simulink model "IEEE_13_BUS_Radial"  (R2021b)
settings: Solver=VariableStepAuto  StartTime=0.0  StopTime=48  RelTol=1e-3
undefined symbols (not defined in the file or in its folder): f611, f632, f633, f634, f645, f646, f650, f652, f671, f675, f680, f684, f692
libraries: simulink x416, slpidlib x13
(part 7 of 7)

== system IEEE_13_BUS_Radial/f675/CONTROLLERS/lPoLC2 ==
  Sum : Sum  Inputs=|++
  base : simulink/Sources/Repeating Sequence Stair  OutValues=f675.PoLC2.l  tsamp=f675.PoLC2.ST  OutMin=[]  OutMax=[]  OutDataTypeStr=double  OutputDataTypeScalingMode=double  OutDataType=fixdt(0,8)  ConRadixGroup=Best Precision: Vector-wise  OutScaling=2^-12
  noise : simulink/Sources/Band-Limited White Noise  Cov=f675.PoLC2.Noise  Ts=f675.PoLC2.NoiseST  seed=f675.PoLC2.NoiseSD
  P : Outport  VectorParamsAs1DForOutWhenUnconnected=off
  wires:
  Sum/1 -> P/1
  noise/1 -> Sum/2
  base/1 -> Sum/1

== system IEEE_13_BUS_Radial/f675/CONTROLLERS/lPoLC3 ==
  Sum : Sum  Inputs=|++
  base : simulink/Sources/Repeating Sequence Stair  OutValues=f675.PoLC3.l  tsamp=f675.PoLC3.ST  OutMin=[]  OutMax=[]  OutDataTypeStr=double  OutputDataTypeScalingMode=double  OutDataType=fixdt(0,8)  ConRadixGroup=Best Precision: Vector-wise  OutScaling=2^-12
  noise : simulink/Sources/Band-Limited White Noise  Cov=f675.PoLC3.Noise  Ts=f675.PoLC3.NoiseST  seed=f675.PoLC3.NoiseSD
  P : Outport  VectorParamsAs1DForOutWhenUnconnected=off
  wires:
  Sum/1 -> P/1
  noise/1 -> Sum/2
  base/1 -> Sum/1

== system IEEE_13_BUS_Radial/f675/CONTROLLERS/lPoLC4 ==
  Sum : Sum  Inputs=|++
  base : simulink/Sources/Repeating Sequence Stair  OutValues=f675.PoLC4.l  tsamp=f675.PoLC4.ST  OutMin=[]  OutMax=[]  OutDataTypeStr=double  OutputDataTypeScalingMode=double  OutDataType=fixdt(0,8)  ConRadixGroup=Best Precision: Vector-wise  OutScaling=2^-12
  noise : simulink/Sources/Band-Limited White Noise  Cov=f675.PoLC4.Noise  Ts=f675.PoLC4.NoiseST  seed=f675.PoLC4.NoiseSD
  P : Outport  VectorParamsAs1DForOutWhenUnconnected=off
  wires:
  Sum/1 -> P/1
  noise/1 -> Sum/2
  base/1 -> Sum/1

== system IEEE_13_BUS_Radial/f675/CONTROLLERS/lPoLC5 ==
  Sum : Sum  Inputs=|++
  base : simulink/Sources/Repeating Sequence Stair  OutValues=f675.PoLC5.l  tsamp=f675.PoLC5.ST  OutMin=[]  OutMax=[]  OutDataTypeStr=double  OutputDataTypeScalingMode=double  OutDataType=fixdt(0,8)  ConRadixGroup=Best Precision: Vector-wise  OutScaling=2^-12
  noise : simulink/Sources/Band-Limited White Noise  Cov=f675.PoLC5.Noise  Ts=f675.PoLC5.NoiseST  seed=f675.PoLC5.NoiseSD
  P : Outport  VectorParamsAs1DForOutWhenUnconnected=off
  wires:
  Sum/1 -> P/1
  noise/1 -> Sum/2
  base/1 -> Sum/1

== system IEEE_13_BUS_Radial/f675/CONTROLLERS/lPoLC6 ==
  Sum : Sum  Inputs=|++
  base : simulink/Sources/Repeating Sequence Stair  OutValues=f675.PoLC6.l  tsamp=f675.PoLC6.ST  OutMin=[]  OutMax=[]  OutDataTypeStr=double  OutputDataTypeScalingMode=double  OutDataType=fixdt(0,8)  ConRadixGroup=Best Precision: Vector-wise  OutScaling=2^-12
  noise : simulink/Sources/Band-Limited White Noise  Cov=f675.PoLC6.Noise  Ts=f675.PoLC6.NoiseST  seed=f675.PoLC6.NoiseSD
  P : Outport  VectorParamsAs1DForOutWhenUnconnected=off
  wires:
  Sum/1 -> P/1
  noise/1 -> Sum/2
  base/1 -> Sum/1

== system IEEE_13_BUS_Radial/f675/CONTROLLERS/lPoLC7 ==
  Sum : Sum  Inputs=|++
  base : simulink/Sources/Repeating Sequence Stair  OutValues=f675.PoLC7.l  tsamp=f675.PoLC7.ST  OutMin=[]  OutMax=[]  OutDataTypeStr=double  OutputDataTypeScalingMode=double  OutDataType=fixdt(0,8)  ConRadixGroup=Best Precision: Vector-wise  OutScaling=2^-12
  noise : simulink/Sources/Band-Limited White Noise  Cov=f675.PoLC7.Noise  Ts=f675.PoLC7.NoiseST  seed=f675.PoLC7.NoiseSD
  P : Outport  VectorParamsAs1DForOutWhenUnconnected=off
  wires:
  Sum/1 -> P/1
  noise/1 -> Sum/2
  base/1 -> Sum/1

== system IEEE_13_BUS_Radial/f675/CONTROLLERS/lPoLC8 ==
  Sum : Sum  Inputs=|++
  base : simulink/Sources/Repeating Sequence Stair  OutValues=f675.PoLC8.l  tsamp=f675.PoLC8.ST  OutMin=[]  OutMax=[]  OutDataTypeStr=double  OutputDataTypeScalingMode=double  OutDataType=fixdt(0,8)  ConRadixGroup=Best Precision: Vector-wise  OutScaling=2^-12
  noise : simulink/Sources/Band-Limited White Noise  Cov=f675.PoLC8.Noise  Ts=f675.PoLC8.NoiseST  seed=f675.PoLC8.NoiseSD
  P : Outport  VectorParamsAs1DForOutWhenUnconnected=off
  wires:
  Sum/1 -> P/1
  noise/1 -> Sum/2
  base/1 -> Sum/1

== system IEEE_13_BUS_Radial/f675/CONTROLLERS/lPoLC9 ==
  Sum : Sum  Inputs=|++
  base : simulink/Sources/Repeating Sequence Stair  OutValues=f675.PoLC9.l  tsamp=f675.PoLC9.ST  OutMin=[]  OutMax=[]  OutDataTypeStr=double  OutputDataTypeScalingMode=double  OutDataType=fixdt(0,8)  ConRadixGroup=Best Precision: Vector-wise  OutScaling=2^-12
  noise : simulink/Sources/Band-Limited White Noise  Cov=f675.PoLC9.Noise  Ts=f675.PoLC9.NoiseST  seed=f675.PoLC9.NoiseSD
  P : Outport  VectorParamsAs1DForOutWhenUnconnected=off
  wires:
  Sum/1 -> P/1
  noise/1 -> Sum/2
  base/1 -> Sum/1

== system IEEE_13_BUS_Radial/f675/OPERATIONS GATEWAY/Agent Communications ==
  Enable : EnablePort
  Constant : Constant  Value=0
  Out1 : Outport  VectorParamsAs1DForOutWhenUnconnected=off
  wires:
  Constant/1 -> Out1/1

== system IEEE_13_BUS_Radial/f680/CONTROLLERS/lPoLC1 ==
  Sum : Sum  Inputs=|++
  base : simulink/Sources/Repeating Sequence Stair  OutValues=f680.PoLC1.l  tsamp=f680.PoLC1.ST  OutMin=[]  OutMax=[]  OutDataTypeStr=double  OutputDataTypeScalingMode=double  OutDataType=fixdt(0,8)  ConRadixGroup=Best Precision: Vector-wise  OutScaling=2^-12
  noise : simulink/Sources/Band-Limited White Noise  Cov=f680.PoLC1.Noise  Ts=f680.PoLC1.NoiseST  seed=f680.PoLC1.NoiseSD
  P : Outport  VectorParamsAs1DForOutWhenUnconnected=off
  wires:
  Sum/1 -> P/1
  noise/1 -> Sum/2
  base/1 -> Sum/1

== system IEEE_13_BUS_Radial/f680/CONTROLLERS/lPoLC10 ==
  Sum : Sum  Inputs=|++
  base : simulink/Sources/Repeating Sequence Stair  OutValues=f680.PoLC10.l  tsamp=f680.PoLC10.ST  OutMin=[]  OutMax=[]  OutDataTypeStr=double  OutputDataTypeScalingMode=double  OutDataType=fixdt(0,8)  ConRadixGroup=Best Precision: Vector-wise  OutScaling=2^-12
  noise : simulink/Sources/Band-Limited White Noise  Cov=f680.PoLC10.Noise  Ts=f680.PoLC10.NoiseST  seed=f680.PoLC10.NoiseSD
  P : Outport  VectorParamsAs1DForOutWhenUnconnected=off
  wires:
  Sum/1 -> P/1
  noise/1 -> Sum/2
  base/1 -> Sum/1

== system IEEE_13_BUS_Radial/f680/CONTROLLERS/lPoLC11 ==
  Sum : Sum  Inputs=|++
  base : simulink/Sources/Repeating Sequence Stair  OutValues=f680.PoLC11.l  tsamp=f680.PoLC11.ST  OutMin=[]  OutMax=[]  OutDataTypeStr=double  OutputDataTypeScalingMode=double  OutDataType=fixdt(0,8)  ConRadixGroup=Best Precision: Vector-wise  OutScaling=2^-12
  noise : simulink/Sources/Band-Limited White Noise  Cov=f680.PoLC11.Noise  Ts=f680.PoLC11.NoiseST  seed=f680.PoLC11.NoiseSD
  P : Outport  VectorParamsAs1DForOutWhenUnconnected=off
  wires:
  Sum/1 -> P/1
  noise/1 -> Sum/2
  base/1 -> Sum/1

== system IEEE_13_BUS_Radial/f680/CONTROLLERS/lPoLC12 ==
  Sum : Sum  Inputs=|++
  base : simulink/Sources/Repeating Sequence Stair  OutValues=f680.PoLC12.l  tsamp=f680.PoLC12.ST  OutMin=[]  OutMax=[]  OutDataTypeStr=double  OutputDataTypeScalingMode=double  OutDataType=fixdt(0,8)  ConRadixGroup=Best Precision: Vector-wise  OutScaling=2^-12
  noise : simulink/Sources/Band-Limited White Noise  Cov=f680.PoLC12.Noise  Ts=f680.PoLC12.NoiseST  seed=f680.PoLC12.NoiseSD
  P : Outport  VectorParamsAs1DForOutWhenUnconnected=off
  wires:
  Sum/1 -> P/1
  noise/1 -> Sum/2
  base/1 -> Sum/1

== system IEEE_13_BUS_Radial/f680/CONTROLLERS/lPoLC13 ==
  Sum : Sum  Inputs=|++
  base : simulink/Sources/Repeating Sequence Stair  OutValues=f680.PoLC13.l  tsamp=f680.PoLC13.ST  OutMin=[]  OutMax=[]  OutDataTypeStr=double  OutputDataTypeScalingMode=double  OutDataType=fixdt(0,8)  ConRadixGroup=Best Precision: Vector-wise  OutScaling=2^-12
  noise : simulink/Sources/Band-Limited White Noise  Cov=f680.PoLC13.Noise  Ts=f680.PoLC13.NoiseST  seed=f680.PoLC13.NoiseSD
  P : Outport  VectorParamsAs1DForOutWhenUnconnected=off
  wires:
  Sum/1 -> P/1
  noise/1 -> Sum/2
  base/1 -> Sum/1

== system IEEE_13_BUS_Radial/f680/CONTROLLERS/lPoLC14 ==
  Sum : Sum  Inputs=|++
  base : simulink/Sources/Repeating Sequence Stair  OutValues=f680.PoLC14.l  tsamp=f680.PoLC14.ST  OutMin=[]  OutMax=[]  OutDataTypeStr=double  OutputDataTypeScalingMode=double  OutDataType=fixdt(0,8)  ConRadixGroup=Best Precision: Vector-wise  OutScaling=2^-12
  noise : simulink/Sources/Band-Limited White Noise  Cov=f680.PoLC14.Noise  Ts=f680.PoLC14.NoiseST  seed=f680.PoLC14.NoiseSD
  P : Outport  VectorParamsAs1DForOutWhenUnconnected=off
  wires:
  Sum/1 -> P/1
  noise/1 -> Sum/2
  base/1 -> Sum/1

== system IEEE_13_BUS_Radial/f680/CONTROLLERS/lPoLC15 ==
  Sum : Sum  Inputs=|++
  base : simulink/Sources/Repeating Sequence Stair  OutValues=f680.PoLC15.l  tsamp=f680.PoLC15.ST  OutMin=[]  OutMax=[]  OutDataTypeStr=double  OutputDataTypeScalingMode=double  OutDataType=fixdt(0,8)  ConRadixGroup=Best Precision: Vector-wise  OutScaling=2^-12
  noise : simulink/Sources/Band-Limited White Noise  Cov=f680.PoLC15.Noise  Ts=f680.PoLC15.NoiseST  seed=f680.PoLC15.NoiseSD
  P : Outport  VectorParamsAs1DForOutWhenUnconnected=off
  wires:
  Sum/1 -> P/1
  noise/1 -> Sum/2
  base/1 -> Sum/1

== system IEEE_13_BUS_Radial/f680/CONTROLLERS/lPoLC16 ==
  cv : Inport
  Sum : Sum  Inputs=|++
  Terminator : Terminator
  base : simulink/Sources/Repeating Sequence Stair  OutValues=f680.PoLC16.l  tsamp=f680.PoLC16.ST  OutMin=[]  OutMax=[]  OutDataTypeStr=double  OutputDataTypeScalingMode=double  OutDataType=fixdt(0,8)  ConRadixGroup=Best Precision: Vector-wise  OutScaling=2^-12
  noise : simulink/Sources/Band-Limited White Noise  Cov=f680.PoLC16.Noise  Ts=f680.PoLC16.NoiseST  seed=f680.PoLC16.NoiseSD
  P : Outport  VectorParamsAs1DForOutWhenUnconnected=off
  wires:
  Sum/1 -> Terminator/1
  noise/1 -> Sum/2
  base/1 -> Sum/1
  cv/1 -> P/1

== system IEEE_13_BUS_Radial/f680/CONTROLLERS/lPoLC2 ==
  Sum : Sum  Inputs=|++
  base : simulink/Sources/Repeating Sequence Stair  OutValues=f680.PoLC2.l  tsamp=f680.PoLC2.ST  OutMin=[]  OutMax=[]  OutDataTypeStr=double  OutputDataTypeScalingMode=double  OutDataType=fixdt(0,8)  ConRadixGroup=Best Precision: Vector-wise  OutScaling=2^-12
  noise : simulink/Sources/Band-Limited White Noise  Cov=f680.PoLC2.Noise  Ts=f680.PoLC2.NoiseST  seed=f680.PoLC2.NoiseSD
  P : Outport  VectorParamsAs1DForOutWhenUnconnected=off
  wires:
  Sum/1 -> P/1
  noise/1 -> Sum/2
  base/1 -> Sum/1

== system IEEE_13_BUS_Radial/f680/CONTROLLERS/lPoLC3 ==
  Sum : Sum  Inputs=|++
  base : simulink/Sources/Repeating Sequence Stair  OutValues=f680.PoLC3.l  tsamp=f680.PoLC3.ST  OutMin=[]  OutMax=[]  OutDataTypeStr=double  OutputDataTypeScalingMode=double  OutDataType=fixdt(0,8)  ConRadixGroup=Best Precision: Vector-wise  OutScaling=2^-12
  noise : simulink/Sources/Band-Limited White Noise  Cov=f680.PoLC3.Noise  Ts=f680.PoLC3.NoiseST  seed=f680.PoLC3.NoiseSD
  P : Outport  VectorParamsAs1DForOutWhenUnconnected=off
  wires:
  Sum/1 -> P/1
  noise/1 -> Sum/2
  base/1 -> Sum/1

== system IEEE_13_BUS_Radial/f680/CONTROLLERS/lPoLC4 ==
  Sum : Sum  Inputs=|++
  base : simulink/Sources/Repeating Sequence Stair  OutValues=f680.PoLC4.l  tsamp=f680.PoLC4.ST  OutMin=[]  OutMax=[]  OutDataTypeStr=double  OutputDataTypeScalingMode=double  OutDataType=fixdt(0,8)  ConRadixGroup=Best Precision: Vector-wise  OutScaling=2^-12
  noise : simulink/Sources/Band-Limited White Noise  Cov=f680.PoLC4.Noise  Ts=f680.PoLC4.NoiseST  seed=f680.PoLC4.NoiseSD
  P : Outport  VectorParamsAs1DForOutWhenUnconnected=off
  wires:
  Sum/1 -> P/1
  noise/1 -> Sum/2
  base/1 -> Sum/1

== system IEEE_13_BUS_Radial/f680/CONTROLLERS/lPoLC5 ==
  Sum : Sum  Inputs=|++
  base : simulink/Sources/Repeating Sequence Stair  OutValues=f680.PoLC5.l  tsamp=f680.PoLC5.ST  OutMin=[]  OutMax=[]  OutDataTypeStr=double  OutputDataTypeScalingMode=double  OutDataType=fixdt(0,8)  ConRadixGroup=Best Precision: Vector-wise  OutScaling=2^-12
  noise : simulink/Sources/Band-Limited White Noise  Cov=f680.PoLC5.Noise  Ts=f680.PoLC5.NoiseST  seed=f680.PoLC5.NoiseSD
  P : Outport  VectorParamsAs1DForOutWhenUnconnected=off
  wires:
  Sum/1 -> P/1
  noise/1 -> Sum/2
  base/1 -> Sum/1

== system IEEE_13_BUS_Radial/f680/CONTROLLERS/lPoLC6 ==
  Sum : Sum  Inputs=|++
  base : simulink/Sources/Repeating Sequence Stair  OutValues=f680.PoLC6.l  tsamp=f680.PoLC6.ST  OutMin=[]  OutMax=[]  OutDataTypeStr=double  OutputDataTypeScalingMode=double  OutDataType=fixdt(0,8)  ConRadixGroup=Best Precision: Vector-wise  OutScaling=2^-12
  noise : simulink/Sources/Band-Limited White Noise  Cov=f680.PoLC6.Noise  Ts=f680.PoLC6.NoiseST  seed=f680.PoLC6.NoiseSD
  P : Outport  VectorParamsAs1DForOutWhenUnconnected=off
  wires:
  Sum/1 -> P/1
  noise/1 -> Sum/2
  base/1 -> Sum/1

== system IEEE_13_BUS_Radial/f680/CONTROLLERS/lPoLC7 ==
  Sum : Sum  Inputs=|++
  base : simulink/Sources/Repeating Sequence Stair  OutValues=f680.PoLC7.l  tsamp=f680.PoLC7.ST  OutMin=[]  OutMax=[]  OutDataTypeStr=double  OutputDataTypeScalingMode=double  OutDataType=fixdt(0,8)  ConRadixGroup=Best Precision: Vector-wise  OutScaling=2^-12
  noise : simulink/Sources/Band-Limited White Noise  Cov=f680.PoLC7.Noise  Ts=f680.PoLC7.NoiseST  seed=f680.PoLC7.NoiseSD
  P : Outport  VectorParamsAs1DForOutWhenUnconnected=off
  wires:
  Sum/1 -> P/1
  noise/1 -> Sum/2
  base/1 -> Sum/1

== system IEEE_13_BUS_Radial/f680/CONTROLLERS/lPoLC8 ==
  Sum : Sum  Inputs=|++
  base : simulink/Sources/Repeating Sequence Stair  OutValues=f680.PoLC8.l  tsamp=f680.PoLC8.ST  OutMin=[]  OutMax=[]  OutDataTypeStr=double  OutputDataTypeScalingMode=double  OutDataType=fixdt(0,8)  ConRadixGroup=Best Precision: Vector-wise  OutScaling=2^-12
  noise : simulink/Sources/Band-Limited White Noise  Cov=f680.PoLC8.Noise  Ts=f680.PoLC8.NoiseST  seed=f680.PoLC8.NoiseSD
  P : Outport  VectorParamsAs1DForOutWhenUnconnected=off
  wires:
  Sum/1 -> P/1
  noise/1 -> Sum/2
  base/1 -> Sum/1

== system IEEE_13_BUS_Radial/f680/CONTROLLERS/lPoLC9 ==
  Sum : Sum  Inputs=|++
  base : simulink/Sources/Repeating Sequence Stair  OutValues=f680.PoLC9.l  tsamp=f680.PoLC9.ST  OutMin=[]  OutMax=[]  OutDataTypeStr=double  OutputDataTypeScalingMode=double  OutDataType=fixdt(0,8)  ConRadixGroup=Best Precision: Vector-wise  OutScaling=2^-12
  noise : simulink/Sources/Band-Limited White Noise  Cov=f680.PoLC9.Noise  Ts=f680.PoLC9.NoiseST  seed=f680.PoLC9.NoiseSD
  P : Outport  VectorParamsAs1DForOutWhenUnconnected=off
  wires:
  Sum/1 -> P/1
  noise/1 -> Sum/2
  base/1 -> Sum/1

== system IEEE_13_BUS_Radial/f680/OPERATIONS GATEWAY/Agent Communications ==
  Enable : EnablePort
  Constant : Constant  Value=0
  Out1 : Outport  VectorParamsAs1DForOutWhenUnconnected=off
  wires:
  Constant/1 -> Out1/1

== system IEEE_13_BUS_Radial/f684/CONTROLLERS/lPoLC1 ==
  Sum : Sum  Inputs=|++
  base : simulink/Sources/Repeating Sequence Stair  OutValues=f684.PoLC1.l  tsamp=f684.PoLC1.ST  OutMin=[]  OutMax=[]  OutDataTypeStr=double  OutputDataTypeScalingMode=double  OutDataType=fixdt(0,8)  ConRadixGroup=Best Precision: Vector-wise  OutScaling=2^-12
  noise : simulink/Sources/Band-Limited White Noise  Cov=f684.PoLC1.Noise  Ts=f684.PoLC1.NoiseST  seed=f684.PoLC1.NoiseSD
  P : Outport  VectorParamsAs1DForOutWhenUnconnected=off
  wires:
  Sum/1 -> P/1
  noise/1 -> Sum/2
  base/1 -> Sum/1

== system IEEE_13_BUS_Radial/f684/CONTROLLERS/lPoLC10 ==
  Sum : Sum  Inputs=|++
  base : simulink/Sources/Repeating Sequence Stair  OutValues=f684.PoLC10.l  tsamp=f684.PoLC10.ST  OutMin=[]  OutMax=[]  OutDataTypeStr=double  OutputDataTypeScalingMode=double  OutDataType=fixdt(0,8)  ConRadixGroup=Best Precision: Vector-wise  OutScaling=2^-12
  noise : simulink/Sources/Band-Limited White Noise  Cov=f684.PoLC10.Noise  Ts=f684.PoLC10.NoiseST  seed=f684.PoLC10.NoiseSD
  P : Outport  VectorParamsAs1DForOutWhenUnconnected=off
  wires:
  Sum/1 -> P/1
  noise/1 -> Sum/2
  base/1 -> Sum/1

== system IEEE_13_BUS_Radial/f684/CONTROLLERS/lPoLC11 ==
  Sum : Sum  Inputs=|++
  base : simulink/Sources/Repeating Sequence Stair  OutValues=f684.PoLC11.l  tsamp=f684.PoLC11.ST  OutMin=[]  OutMax=[]  OutDataTypeStr=double  OutputDataTypeScalingMode=double  OutDataType=fixdt(0,8)  ConRadixGroup=Best Precision: Vector-wise  OutScaling=2^-12
  noise : simulink/Sources/Band-Limited White Noise  Cov=f684.PoLC11.Noise  Ts=f684.PoLC11.NoiseST  seed=f684.PoLC11.NoiseSD
  P : Outport  VectorParamsAs1DForOutWhenUnconnected=off
  wires:
  Sum/1 -> P/1
  noise/1 -> Sum/2
  base/1 -> Sum/1

== system IEEE_13_BUS_Radial/f684/CONTROLLERS/lPoLC12 ==
  Sum : Sum  Inputs=|++
  base : simulink/Sources/Repeating Sequence Stair  OutValues=f684.PoLC12.l  tsamp=f684.PoLC12.ST  OutMin=[]  OutMax=[]  OutDataTypeStr=double  OutputDataTypeScalingMode=double  OutDataType=fixdt(0,8)  ConRadixGroup=Best Precision: Vector-wise  OutScaling=2^-12
  noise : simulink/Sources/Band-Limited White Noise  Cov=f684.PoLC12.Noise  Ts=f684.PoLC12.NoiseST  seed=f684.PoLC12.NoiseSD
  P : Outport  VectorParamsAs1DForOutWhenUnconnected=off
  wires:
  Sum/1 -> P/1
  noise/1 -> Sum/2
  base/1 -> Sum/1

== system IEEE_13_BUS_Radial/f684/CONTROLLERS/lPoLC13 ==
  Sum : Sum  Inputs=|++
  base : simulink/Sources/Repeating Sequence Stair  OutValues=f684.PoLC13.l  tsamp=f684.PoLC13.ST  OutMin=[]  OutMax=[]  OutDataTypeStr=double  OutputDataTypeScalingMode=double  OutDataType=fixdt(0,8)  ConRadixGroup=Best Precision: Vector-wise  OutScaling=2^-12
  noise : simulink/Sources/Band-Limited White Noise  Cov=f684.PoLC13.Noise  Ts=f684.PoLC13.NoiseST  seed=f684.PoLC13.NoiseSD
  P : Outport  VectorParamsAs1DForOutWhenUnconnected=off
  wires:
  Sum/1 -> P/1
  noise/1 -> Sum/2
  base/1 -> Sum/1

== system IEEE_13_BUS_Radial/f684/CONTROLLERS/lPoLC14 ==
  Sum : Sum  Inputs=|++
  base : simulink/Sources/Repeating Sequence Stair  OutValues=f684.PoLC14.l  tsamp=f684.PoLC14.ST  OutMin=[]  OutMax=[]  OutDataTypeStr=double  OutputDataTypeScalingMode=double  OutDataType=fixdt(0,8)  ConRadixGroup=Best Precision: Vector-wise  OutScaling=2^-12
  noise : simulink/Sources/Band-Limited White Noise  Cov=f684.PoLC14.Noise  Ts=f684.PoLC14.NoiseST  seed=f684.PoLC14.NoiseSD
  P : Outport  VectorParamsAs1DForOutWhenUnconnected=off
  wires:
  Sum/1 -> P/1
  noise/1 -> Sum/2
  base/1 -> Sum/1

== system IEEE_13_BUS_Radial/f684/CONTROLLERS/lPoLC15 ==
  Sum : Sum  Inputs=|++
  base : simulink/Sources/Repeating Sequence Stair  OutValues=f684.PoLC15.l  tsamp=f684.PoLC15.ST  OutMin=[]  OutMax=[]  OutDataTypeStr=double  OutputDataTypeScalingMode=double  OutDataType=fixdt(0,8)  ConRadixGroup=Best Precision: Vector-wise  OutScaling=2^-12
  noise : simulink/Sources/Band-Limited White Noise  Cov=f684.PoLC15.Noise  Ts=f684.PoLC15.NoiseST  seed=f684.PoLC15.NoiseSD
  P : Outport  VectorParamsAs1DForOutWhenUnconnected=off
  wires:
  Sum/1 -> P/1
  noise/1 -> Sum/2
  base/1 -> Sum/1

== system IEEE_13_BUS_Radial/f684/CONTROLLERS/lPoLC16 ==
  cv : Inport
  Sum : Sum  Inputs=|++
  Terminator : Terminator
  base : simulink/Sources/Repeating Sequence Stair  OutValues=f684.PoLC16.l  tsamp=f684.PoLC16.ST  OutMin=[]  OutMax=[]  OutDataTypeStr=double  OutputDataTypeScalingMode=double  OutDataType=fixdt(0,8)  ConRadixGroup=Best Precision: Vector-wise  OutScaling=2^-12
  noise : simulink/Sources/Band-Limited White Noise  Cov=f684.PoLC16.Noise  Ts=f684.PoLC16.NoiseST  seed=f684.PoLC16.NoiseSD
  P : Outport  VectorParamsAs1DForOutWhenUnconnected=off
  wires:
  Sum/1 -> Terminator/1
  noise/1 -> Sum/2
  base/1 -> Sum/1
  cv/1 -> P/1

== system IEEE_13_BUS_Radial/f684/CONTROLLERS/lPoLC2 ==
  Sum : Sum  Inputs=|++
  base : simulink/Sources/Repeating Sequence Stair  OutValues=f684.PoLC2.l  tsamp=f684.PoLC2.ST  OutMin=[]  OutMax=[]  OutDataTypeStr=double  OutputDataTypeScalingMode=double  OutDataType=fixdt(0,8)  ConRadixGroup=Best Precision: Vector-wise  OutScaling=2^-12
  noise : simulink/Sources/Band-Limited White Noise  Cov=f684.PoLC2.Noise  Ts=f684.PoLC2.NoiseST  seed=f684.PoLC2.NoiseSD
  P : Outport  VectorParamsAs1DForOutWhenUnconnected=off
  wires:
  Sum/1 -> P/1
  noise/1 -> Sum/2
  base/1 -> Sum/1

== system IEEE_13_BUS_Radial/f684/CONTROLLERS/lPoLC3 ==
  Sum : Sum  Inputs=|++
  base : simulink/Sources/Repeating Sequence Stair  OutValues=f684.PoLC3.l  tsamp=f684.PoLC3.ST  OutMin=[]  OutMax=[]  OutDataTypeStr=double  OutputDataTypeScalingMode=double  OutDataType=fixdt(0,8)  ConRadixGroup=Best Precision: Vector-wise  OutScaling=2^-12
  noise : simulink/Sources/Band-Limited White Noise  Cov=f684.PoLC3.Noise  Ts=f684.PoLC3.NoiseST  seed=f684.PoLC3.NoiseSD
  P : Outport  VectorParamsAs1DForOutWhenUnconnected=off
  wires:
  Sum/1 -> P/1
  noise/1 -> Sum/2
  base/1 -> Sum/1

== system IEEE_13_BUS_Radial/f684/CONTROLLERS/lPoLC4 ==
  Sum : Sum  Inputs=|++
  base : simulink/Sources/Repeating Sequence Stair  OutValues=f684.PoLC4.l  tsamp=f684.PoLC4.ST  OutMin=[]  OutMax=[]  OutDataTypeStr=double  OutputDataTypeScalingMode=double  OutDataType=fixdt(0,8)  ConRadixGroup=Best Precision: Vector-wise  OutScaling=2^-12
  noise : simulink/Sources/Band-Limited White Noise  Cov=f684.PoLC4.Noise  Ts=f684.PoLC4.NoiseST  seed=f684.PoLC4.NoiseSD
  P : Outport  VectorParamsAs1DForOutWhenUnconnected=off
  wires:
  Sum/1 -> P/1
  noise/1 -> Sum/2
  base/1 -> Sum/1

== system IEEE_13_BUS_Radial/f684/CONTROLLERS/lPoLC5 ==
  Sum : Sum  Inputs=|++
  base : simulink/Sources/Repeating Sequence Stair  OutValues=f684.PoLC5.l  tsamp=f684.PoLC5.ST  OutMin=[]  OutMax=[]  OutDataTypeStr=double  OutputDataTypeScalingMode=double  OutDataType=fixdt(0,8)  ConRadixGroup=Best Precision: Vector-wise  OutScaling=2^-12
  noise : simulink/Sources/Band-Limited White Noise  Cov=f684.PoLC5.Noise  Ts=f684.PoLC5.NoiseST  seed=f684.PoLC5.NoiseSD
  P : Outport  VectorParamsAs1DForOutWhenUnconnected=off
  wires:
  Sum/1 -> P/1
  noise/1 -> Sum/2
  base/1 -> Sum/1

== system IEEE_13_BUS_Radial/f684/CONTROLLERS/lPoLC6 ==
  Sum : Sum  Inputs=|++
  base : simulink/Sources/Repeating Sequence Stair  OutValues=f684.PoLC6.l  tsamp=f684.PoLC6.ST  OutMin=[]  OutMax=[]  OutDataTypeStr=double  OutputDataTypeScalingMode=double  OutDataType=fixdt(0,8)  ConRadixGroup=Best Precision: Vector-wise  OutScaling=2^-12
  noise : simulink/Sources/Band-Limited White Noise  Cov=f684.PoLC6.Noise  Ts=f684.PoLC6.NoiseST  seed=f684.PoLC6.NoiseSD
  P : Outport  VectorParamsAs1DForOutWhenUnconnected=off
  wires:
  Sum/1 -> P/1
  noise/1 -> Sum/2
  base/1 -> Sum/1

== system IEEE_13_BUS_Radial/f684/CONTROLLERS/lPoLC7 ==
  Sum : Sum  Inputs=|++
  base : simulink/Sources/Repeating Sequence Stair  OutValues=f684.PoLC7.l  tsamp=f684.PoLC7.ST  OutMin=[]  OutMax=[]  OutDataTypeStr=double  OutputDataTypeScalingMode=double  OutDataType=fixdt(0,8)  ConRadixGroup=Best Precision: Vector-wise  OutScaling=2^-12
  noise : simulink/Sources/Band-Limited White Noise  Cov=f684.PoLC7.Noise  Ts=f684.PoLC7.NoiseST  seed=f684.PoLC7.NoiseSD
  P : Outport  VectorParamsAs1DForOutWhenUnconnected=off
  wires:
  Sum/1 -> P/1
  noise/1 -> Sum/2
  base/1 -> Sum/1

== system IEEE_13_BUS_Radial/f684/CONTROLLERS/lPoLC8 ==
  Sum : Sum  Inputs=|++
  base : simulink/Sources/Repeating Sequence Stair  OutValues=f684.PoLC8.l  tsamp=f684.PoLC8.ST  OutMin=[]  OutMax=[]  OutDataTypeStr=double  OutputDataTypeScalingMode=double  OutDataType=fixdt(0,8)  ConRadixGroup=Best Precision: Vector-wise  OutScaling=2^-12
  noise : simulink/Sources/Band-Limited White Noise  Cov=f684.PoLC8.Noise  Ts=f684.PoLC8.NoiseST  seed=f684.PoLC8.NoiseSD
  P : Outport  VectorParamsAs1DForOutWhenUnconnected=off
  wires:
  Sum/1 -> P/1
  noise/1 -> Sum/2
  base/1 -> Sum/1

== system IEEE_13_BUS_Radial/f684/CONTROLLERS/lPoLC9 ==
  Sum : Sum  Inputs=|++
  base : simulink/Sources/Repeating Sequence Stair  OutValues=f684.PoLC9.l  tsamp=f684.PoLC9.ST  OutMin=[]  OutMax=[]  OutDataTypeStr=double  OutputDataTypeScalingMode=double  OutDataType=fixdt(0,8)  ConRadixGroup=Best Precision: Vector-wise  OutScaling=2^-12
  noise : simulink/Sources/Band-Limited White Noise  Cov=f684.PoLC9.Noise  Ts=f684.PoLC9.NoiseST  seed=f684.PoLC9.NoiseSD
  P : Outport  VectorParamsAs1DForOutWhenUnconnected=off
  wires:
  Sum/1 -> P/1
  noise/1 -> Sum/2
  base/1 -> Sum/1

== system IEEE_13_BUS_Radial/f684/OPERATIONS GATEWAY/Agent Communications ==
  Enable : EnablePort
  Constant : Constant  Value=0
  Out1 : Outport  VectorParamsAs1DForOutWhenUnconnected=off
  wires:
  Constant/1 -> Out1/1

== system IEEE_13_BUS_Radial/f692/CONTROLLERS/lPoLC1 ==
  Sum : Sum  Inputs=|++
  base : simulink/Sources/Repeating Sequence Stair  OutValues=f692.PoLC1.l  tsamp=f692.PoLC1.ST  OutMin=[]  OutMax=[]  OutDataTypeStr=double  OutputDataTypeScalingMode=double  OutDataType=fixdt(0,8)  ConRadixGroup=Best Precision: Vector-wise  OutScaling=2^-12
  noise : simulink/Sources/Band-Limited White Noise  Cov=f692.PoLC1.Noise  Ts=f692.PoLC1.NoiseST  seed=f692.PoLC1.NoiseSD
  P : Outport  VectorParamsAs1DForOutWhenUnconnected=off
  wires:
  Sum/1 -> P/1
  noise/1 -> Sum/2
  base/1 -> Sum/1

== system IEEE_13_BUS_Radial/f692/CONTROLLERS/lPoLC10 ==
  Sum : Sum  Inputs=|++
  base : simulink/Sources/Repeating Sequence Stair  OutValues=f692.PoLC10.l  tsamp=f692.PoLC10.ST  OutMin=[]  OutMax=[]  OutDataTypeStr=double  OutputDataTypeScalingMode=double  OutDataType=fixdt(0,8)  ConRadixGroup=Best Precision: Vector-wise  OutScaling=2^-12
  noise : simulink/Sources/Band-Limited White Noise  Cov=f692.PoLC10.Noise  Ts=f692.PoLC10.NoiseST  seed=f692.PoLC10.NoiseSD
  P : Outport  VectorParamsAs1DForOutWhenUnconnected=off
  wires:
  Sum/1 -> P/1
  noise/1 -> Sum/2
  base/1 -> Sum/1

== system IEEE_13_BUS_Radial/f692/CONTROLLERS/lPoLC11 ==
  Sum : Sum  Inputs=|++
  base : simulink/Sources/Repeating Sequence Stair  OutValues=f692.PoLC11.l  tsamp=f692.PoLC11.ST  OutMin=[]  OutMax=[]  OutDataTypeStr=double  OutputDataTypeScalingMode=double  OutDataType=fixdt(0,8)  ConRadixGroup=Best Precision: Vector-wise  OutScaling=2^-12
  noise : simulink/Sources/Band-Limited White Noise  Cov=f692.PoLC11.Noise  Ts=f692.PoLC11.NoiseST  seed=f692.PoLC11.NoiseSD
  P : Outport  VectorParamsAs1DForOutWhenUnconnected=off
  wires:
  Sum/1 -> P/1
  noise/1 -> Sum/2
  base/1 -> Sum/1

== system IEEE_13_BUS_Radial/f692/CONTROLLERS/lPoLC12 ==
  Sum : Sum  Inputs=|++
  base : simulink/Sources/Repeating Sequence Stair  OutValues=f692.PoLC12.l  tsamp=f692.PoLC12.ST  OutMin=[]  OutMax=[]  OutDataTypeStr=double  OutputDataTypeScalingMode=double  OutDataType=fixdt(0,8)  ConRadixGroup=Best Precision: Vector-wise  OutScaling=2^-12
  noise : simulink/Sources/Band-Limited White Noise  Cov=f692.PoLC12.Noise  Ts=f692.PoLC12.NoiseST  seed=f692.PoLC12.NoiseSD
  P : Outport  VectorParamsAs1DForOutWhenUnconnected=off
  wires:
  Sum/1 -> P/1
  noise/1 -> Sum/2
  base/1 -> Sum/1

== system IEEE_13_BUS_Radial/f692/CONTROLLERS/lPoLC13 ==
  Sum : Sum  Inputs=|++
  base : simulink/Sources/Repeating Sequence Stair  OutValues=f692.PoLC13.l  tsamp=f692.PoLC13.ST  OutMin=[]  OutMax=[]  OutDataTypeStr=double  OutputDataTypeScalingMode=double  OutDataType=fixdt(0,8)  ConRadixGroup=Best Precision: Vector-wise  OutScaling=2^-12
  noise : simulink/Sources/Band-Limited White Noise  Cov=f692.PoLC13.Noise  Ts=f692.PoLC13.NoiseST  seed=f692.PoLC13.NoiseSD
  P : Outport  VectorParamsAs1DForOutWhenUnconnected=off
  wires:
  Sum/1 -> P/1
  noise/1 -> Sum/2
  base/1 -> Sum/1

== system IEEE_13_BUS_Radial/f692/CONTROLLERS/lPoLC14 ==
  Sum : Sum  Inputs=|++
  base : simulink/Sources/Repeating Sequence Stair  OutValues=f692.PoLC14.l  tsamp=f692.PoLC14.ST  OutMin=[]  OutMax=[]  OutDataTypeStr=double  OutputDataTypeScalingMode=double  OutDataType=fixdt(0,8)  ConRadixGroup=Best Precision: Vector-wise  OutScaling=2^-12
  noise : simulink/Sources/Band-Limited White Noise  Cov=f692.PoLC14.Noise  Ts=f692.PoLC14.NoiseST  seed=f692.PoLC14.NoiseSD
  P : Outport  VectorParamsAs1DForOutWhenUnconnected=off
  wires:
  Sum/1 -> P/1
  noise/1 -> Sum/2
  base/1 -> Sum/1

== system IEEE_13_BUS_Radial/f692/CONTROLLERS/lPoLC15 ==
  Sum : Sum  Inputs=|++
  base : simulink/Sources/Repeating Sequence Stair  OutValues=f692.PoLC15.l  tsamp=f692.PoLC15.ST  OutMin=[]  OutMax=[]  OutDataTypeStr=double  OutputDataTypeScalingMode=double  OutDataType=fixdt(0,8)  ConRadixGroup=Best Precision: Vector-wise  OutScaling=2^-12
  noise : simulink/Sources/Band-Limited White Noise  Cov=f692.PoLC15.Noise  Ts=f692.PoLC15.NoiseST  seed=f692.PoLC15.NoiseSD
  P : Outport  VectorParamsAs1DForOutWhenUnconnected=off
  wires:
  Sum/1 -> P/1
  noise/1 -> Sum/2
  base/1 -> Sum/1

== system IEEE_13_BUS_Radial/f692/CONTROLLERS/lPoLC16 ==
  cv : Inport
  Sum : Sum  Inputs=|++
  Terminator : Terminator
  base : simulink/Sources/Repeating Sequence Stair  OutValues=f692.PoLC16.l  tsamp=f692.PoLC16.ST  OutMin=[]  OutMax=[]  OutDataTypeStr=double  OutputDataTypeScalingMode=double  OutDataType=fixdt(0,8)  ConRadixGroup=Best Precision: Vector-wise  OutScaling=2^-12
  noise : simulink/Sources/Band-Limited White Noise  Cov=f692.PoLC16.Noise  Ts=f692.PoLC16.NoiseST  seed=f692.PoLC16.NoiseSD
  P : Outport  VectorParamsAs1DForOutWhenUnconnected=off
  wires:
  Sum/1 -> Terminator/1
  noise/1 -> Sum/2
  base/1 -> Sum/1
  cv/1 -> P/1

== system IEEE_13_BUS_Radial/f692/CONTROLLERS/lPoLC2 ==
  Sum : Sum  Inputs=|++
  base : simulink/Sources/Repeating Sequence Stair  OutValues=f692.PoLC2.l  tsamp=f692.PoLC2.ST  OutMin=[]  OutMax=[]  OutDataTypeStr=double  OutputDataTypeScalingMode=double  OutDataType=fixdt(0,8)  ConRadixGroup=Best Precision: Vector-wise  OutScaling=2^-12
  noise : simulink/Sources/Band-Limited White Noise  Cov=f692.PoLC2.Noise  Ts=f692.PoLC2.NoiseST  seed=f692.PoLC2.NoiseSD
  P : Outport  VectorParamsAs1DForOutWhenUnconnected=off
  wires:
  Sum/1 -> P/1
  noise/1 -> Sum/2
  base/1 -> Sum/1

== system IEEE_13_BUS_Radial/f692/CONTROLLERS/lPoLC3 ==
  Sum : Sum  Inputs=|++
  base : simulink/Sources/Repeating Sequence Stair  OutValues=f692.PoLC3.l  tsamp=f692.PoLC3.ST  OutMin=[]  OutMax=[]  OutDataTypeStr=double  OutputDataTypeScalingMode=double  OutDataType=fixdt(0,8)  ConRadixGroup=Best Precision: Vector-wise  OutScaling=2^-12
  noise : simulink/Sources/Band-Limited White Noise  Cov=f692.PoLC3.Noise  Ts=f692.PoLC3.NoiseST  seed=f692.PoLC3.NoiseSD
  P : Outport  VectorParamsAs1DForOutWhenUnconnected=off
  wires:
  Sum/1 -> P/1
  noise/1 -> Sum/2
  base/1 -> Sum/1

== system IEEE_13_BUS_Radial/f692/CONTROLLERS/lPoLC4 ==
  Sum : Sum  Inputs=|++
  base : simulink/Sources/Repeating Sequence Stair  OutValues=f692.PoLC4.l  tsamp=f692.PoLC4.ST  OutMin=[]  OutMax=[]  OutDataTypeStr=double  OutputDataTypeScalingMode=double  OutDataType=fixdt(0,8)  ConRadixGroup=Best Precision: Vector-wise  OutScaling=2^-12
  noise : simulink/Sources/Band-Limited White Noise  Cov=f692.PoLC4.Noise  Ts=f692.PoLC4.NoiseST  seed=f692.PoLC4.NoiseSD
  P : Outport  VectorParamsAs1DForOutWhenUnconnected=off
  wires:
  Sum/1 -> P/1
  noise/1 -> Sum/2
  base/1 -> Sum/1

== system IEEE_13_BUS_Radial/f692/CONTROLLERS/lPoLC5 ==
  Sum : Sum  Inputs=|++
  base : simulink/Sources/Repeating Sequence Stair  OutValues=f692.PoLC5.l  tsamp=f692.PoLC5.ST  OutMin=[]  OutMax=[]  OutDataTypeStr=double  OutputDataTypeScalingMode=double  OutDataType=fixdt(0,8)  ConRadixGroup=Best Precision: Vector-wise  OutScaling=2^-12
  noise : simulink/Sources/Band-Limited White Noise  Cov=f692.PoLC5.Noise  Ts=f692.PoLC5.NoiseST  seed=f692.PoLC5.NoiseSD
  P : Outport  VectorParamsAs1DForOutWhenUnconnected=off
  wires:
  Sum/1 -> P/1
  noise/1 -> Sum/2
  base/1 -> Sum/1

== system IEEE_13_BUS_Radial/f692/CONTROLLERS/lPoLC6 ==
  Sum : Sum  Inputs=|++
  base : simulink/Sources/Repeating Sequence Stair  OutValues=f692.PoLC6.l  tsamp=f692.PoLC6.ST  OutMin=[]  OutMax=[]  OutDataTypeStr=double  OutputDataTypeScalingMode=double  OutDataType=fixdt(0,8)  ConRadixGroup=Best Precision: Vector-wise  OutScaling=2^-12
  noise : simulink/Sources/Band-Limited White Noise  Cov=f692.PoLC6.Noise  Ts=f692.PoLC6.NoiseST  seed=f692.PoLC6.NoiseSD
  P : Outport  VectorParamsAs1DForOutWhenUnconnected=off
  wires:
  Sum/1 -> P/1
  noise/1 -> Sum/2
  base/1 -> Sum/1

== system IEEE_13_BUS_Radial/f692/CONTROLLERS/lPoLC7 ==
  Sum : Sum  Inputs=|++
  base : simulink/Sources/Repeating Sequence Stair  OutValues=f692.PoLC7.l  tsamp=f692.PoLC7.ST  OutMin=[]  OutMax=[]  OutDataTypeStr=double  OutputDataTypeScalingMode=double  OutDataType=fixdt(0,8)  ConRadixGroup=Best Precision: Vector-wise  OutScaling=2^-12
  noise : simulink/Sources/Band-Limited White Noise  Cov=f692.PoLC7.Noise  Ts=f692.PoLC7.NoiseST  seed=f692.PoLC7.NoiseSD
  P : Outport  VectorParamsAs1DForOutWhenUnconnected=off
  wires:
  Sum/1 -> P/1
  noise/1 -> Sum/2
  base/1 -> Sum/1

== system IEEE_13_BUS_Radial/f692/CONTROLLERS/lPoLC8 ==
  Sum : Sum  Inputs=|++
  base : simulink/Sources/Repeating Sequence Stair  OutValues=f692.PoLC8.l  tsamp=f692.PoLC8.ST  OutMin=[]  OutMax=[]  OutDataTypeStr=double  OutputDataTypeScalingMode=double  OutDataType=fixdt(0,8)  ConRadixGroup=Best Precision: Vector-wise  OutScaling=2^-12
  noise : simulink/Sources/Band-Limited White Noise  Cov=f692.PoLC8.Noise  Ts=f692.PoLC8.NoiseST  seed=f692.PoLC8.NoiseSD
  P : Outport  VectorParamsAs1DForOutWhenUnconnected=off
  wires:
  Sum/1 -> P/1
  noise/1 -> Sum/2
  base/1 -> Sum/1

== system IEEE_13_BUS_Radial/f692/CONTROLLERS/lPoLC9 ==
  Sum : Sum  Inputs=|++
  base : simulink/Sources/Repeating Sequence Stair  OutValues=f692.PoLC9.l  tsamp=f692.PoLC9.ST  OutMin=[]  OutMax=[]  OutDataTypeStr=double  OutputDataTypeScalingMode=double  OutDataType=fixdt(0,8)  ConRadixGroup=Best Precision: Vector-wise  OutScaling=2^-12
  noise : simulink/Sources/Band-Limited White Noise  Cov=f692.PoLC9.Noise  Ts=f692.PoLC9.NoiseST  seed=f692.PoLC9.NoiseSD
  P : Outport  VectorParamsAs1DForOutWhenUnconnected=off
  wires:
  Sum/1 -> P/1
  noise/1 -> Sum/2
  base/1 -> Sum/1

== system IEEE_13_BUS_Radial/f692/OPERATIONS GATEWAY/Agent Communications ==
  Enable : EnablePort
  Constant : Constant  Value=0
  Out1 : Outport  VectorParamsAs1DForOutWhenUnconnected=off
  wires:
  Constant/1 -> Out1/1
